simulink model "ECE551_proj1"  (R2018a)
settings: Solver=VariableStepAuto  StartTime=0.0  StopTime=0.03  RelTol=1e-3
values from neighbouring files (symbols this model uses):
  A = d*A1+d1*A2    [269_1.m]    (also in DifRelFil.m = (2/Nsc)*cos(2*pi*n/Nsc); DigiDiffRelay.m = (2/Nsc)*cos(2*pi*n/Nsc); DigiRelay.m = (2/Nsc)*cos(2*pi*n/Nsc); DigiRelay2.m = (2/Nsc)*cos(2*pi*n/Nsc))
  B = d*B1+d1*B2    [269_1.m]    (also in DifRelFil.m = (2/Nsc)*sin(2*pi*n/Nsc); DigiDiffRelay.m = (2/Nsc)*sin(2*pi*n/Nsc); DigiRelay.m = (2/Nsc)*sin(2*pi*n/Nsc); DigiRelay2.m = (2/Nsc)*sin(2*pi*n/Nsc))
  Bd = (A1−A2)*X    [269_1.m]    (also in ECE551_Project_part1.m = (A1-A2)*X; ECE551_Project_part2.m = (A1-A2)*X)
  C = d*C1+d1*C2    [269_1.m]    (also in ECE347HW5.m = Yc*(1 + Z*Yc/4); ECE545HW6.m = 0.001; ECE551HW1.m = 0.0001; ECE551_Project_part1.m)
settings Model: Creator=clarke6  LastModifiedBy=clarke6

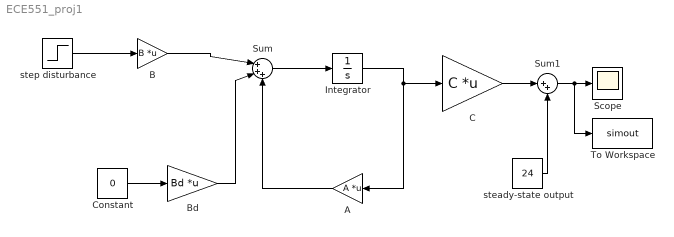
== system ECE551_proj1 ==
  A : Gain  Gain=A  Multiplication=Matrix(K*u)
  B : Gain  Gain=B  Multiplication=Matrix(K*u)
  Bd : Gain  Gain=Bd  Multiplication=Matrix(K*u)
  C : Gain  Gain=C  Multiplication=Matrix(K*u)
  Constant : Constant  Value=0
  Integrator : Integrator
  Scope : Scope
  Sum : Sum  Inputs=|+++
  Sum1 : Sum  Inputs=|++
  To Workspace : ToWorkspace  VariableName=simout  SaveFormat=Timeseries  SampleTime=-1
  steady-state output : Constant  Value=24
  step disturbance : Step  Time=0  SampleTime=0
  wires:
  B/1 -> Sum/1
  Bd/1 -> Sum/2
  A/1 -> Sum/3
  Sum/1 -> Integrator/1
  Integrator/1 -> A/1, C/1
  step disturbance/1 -> B/1
  Sum1/1 -> To Workspace/1, Scope/1
  C/1 -> Sum1/1
  Constant/1 -> Bd/1
  steady-state output/1 -> Sum1/2
